simulink model "Part3og"  (R2019b)
settings: Solver=VariableStepAuto  StartTime=0.0  StopTime=10.0  RelTol=1e-3
settings Model: Creator=Russty  LastModifiedBy=TimRo
settings DataIOCC: ReturnWorkspaceOutputs=off
settings DebuggingCC: ArithmeticOperatorsInVariantConditions=warning
settings SFSimCC: CustomCodeUndefinedFunction=UseInterfaceOnly

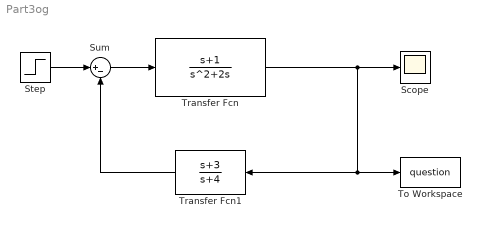
== system Part3og ==
  Scope : Scope
  Step : Step  Time=0  SampleTime=0.001
  Sum : Sum  Inputs=|+-
  To Workspace : ToWorkspace  VariableName=question  SaveFormat=Timeseries  SampleTime=-1
  Transfer Fcn : TransferFcn  Numerator=[1, 1]  Denominator=[1, 2, 0]
  Transfer Fcn1 : TransferFcn  Numerator=[1, 3]  Denominator=[1 4]
  wires:
  Transfer Fcn/1 -> Scope/1, Transfer Fcn1/1, To Workspace/1
  Transfer Fcn1/1 -> Sum/2
  Sum/1 -> Transfer Fcn/1
  Step/1 -> Sum/1
